simulink model "DiffEq1_Model"  (R2025b)
settings: Solver=FixedStepDiscrete  StartTime=0.0  StopTime=20  FixedStep=1  RelTol=1e-3
settings Model: Creator=Rashid  LastModifiedBy=Rashid

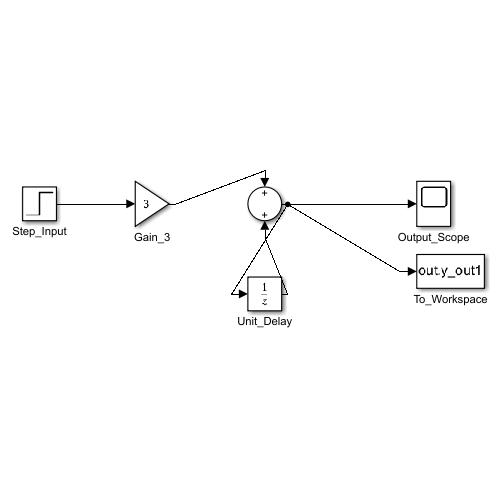
[thumbnail: Simulink's stored preview of the top-level diagram]
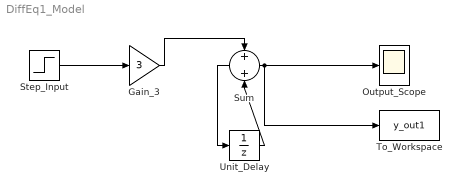
== system DiffEq1_Model ==
  Gain_3 : Gain  Gain=3
  Output_Scope : Scope
  Step_Input : Step  Time=0  SampleTime=0
  Sum : Sum
  To_Workspace : ToWorkspace  VariableName=y_out1  SampleTime=-1
  Unit_Delay : UnitDelay  HasFrameUpgradeWarning=on
  wires:
  Step_Input/1 -> Gain_3/1
  Gain_3/1 -> Sum/1
  Sum/1 -> Output_Scope/1, Unit_Delay/1, To_Workspace/1
  Unit_Delay/1 -> Sum/2
